simulink library "Simulation_lib"  (R2023b)
settings: Solver=VariableStepAuto  StartTime=0.0  StopTime=10.0  RelTol=1e-3
undefined symbols (not defined in the file): X, Y, Z
libraries: sm_lib x48, $bdroot x18, nesl_utility x16, fl_lib x15, ee_lib x3, simulink_extras x1
(part 3 of 3)

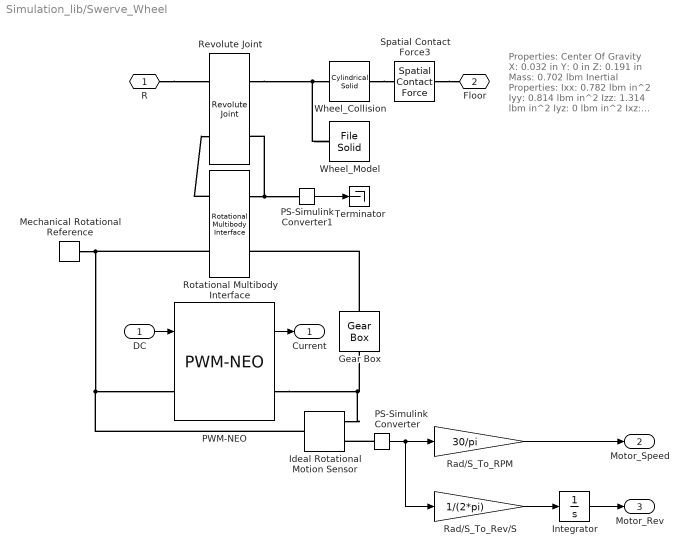
== system Simulation_lib/Swerve_Wheel ==
  note: Properties:
      | Center Of Gravity
      | X: 0.032 in
      | Y: 0 in
      | Z: 0.191 in
      | Mass: 0.702 lbm
      | Inertial Properties:
      | Ixx: 0.782 lbm in^2
      | Iyy: 0.814 lbm in^2
      | Izz: 1.314 lbm in^2
      | Iyz: 0 lbm in^2
      | Ixz: 0.004 lbm in^2
      | Ixy: 0 lbm in^2
      | Cut & Paste:
      | 0.702
      | [0.032 0 0.191]
      | [0.782 0.814 1.314]
      | [0 0.004 0]
  DC : Inport
  Gear Box : fl_lib/Mechanical/Mechanisms/Gear Box  ratio=8.14  t_in_specify=off  t_in_priority=None  t_in=0 N*m  t_in_nominal_specify=off  t_in_nominal_unit=N*m  t_in_nominal_value=1  t_out_specify=off  t_out_priority=None  t_out=0 N*m  t_out_nominal_specify=off  t_out_nominal_unit=N*m  t_out_nominal_value=1
  Ideal Rotational Motion Sensor : fl_lib/Mechanical/Mechanical Sensors/Ideal Rotational Motion Sensor  reference=foundation.enum.MeasurementReference.difference  acceleration_port=false  velocity_port=true  position_port=false  wrap_angle=false  offset=0 rad
      settings: InternalSimscapePortConfiguration="{\"Bottom\":[],\"Left\":[{\"id\":\"R\",\"label\":\"R\",\"type\":\"foundation.mechanical.rotational.rotational\"}],\"Right\":[{\"id\":\"C\",\"label\":\"C\",\"type\":\"foundation.mechanical.rotational.rotational\"},{\"id\":\"W\",\"label\":\"W\",\"type\":\"output\"}],\"Top\":[]}"
  Integrator : Integrator
  Mechanical Rotational Reference : fl_lib/Mechanical/Rotational Elements/Mechanical Rotational Reference
  PS-Simulink Converter : nesl_utility/PS-Simulink Converter  PhysicalDomain=network_engine_domain  SubClassName=ps_output  LeftPortType=input  RightPortType=output  PseudoPeriodic=off  Frequencies=[]  VectorFormat=inherit  Unit=inherit  AffineConversion=off
  PS-Simulink Converter1 : nesl_utility/PS-Simulink Converter  PhysicalDomain=network_engine_domain  SubClassName=ps_output  LeftPortType=input  RightPortType=output  PseudoPeriodic=off  Frequencies=[]  VectorFormat=inherit  Unit=inherit  AffineConversion=off
  PWM-NEO : $bdroot/PWM-NEO  SystemSampleTime=-1  VariantActivationTime=update diagram  AllowFlexibleInterface=on  Latency=0  AutoFrameSizeCalculation=off
  Rad/S_To_RPM : Gain  Gain=30/pi
  Rad/S_To_Rev/S : Gain  Gain=1/(2*pi)
  Revolute Joint : sm_lib/Joints/Revolute Joint  JointMode=Normal  SenseConstraintForce=off  SenseConstraintForceX=off  SenseConstraintForceY=off  SenseConstraintForceZ=off  SenseConstraintTorque=off  SenseConstraintTorqueX=off  SenseConstraintTorqueY=off  SenseConstraintTorqueZ=off  SenseTotalForce=off  SenseTotalForceX=off  SenseTotalForceY=off  SenseTotalForceZ=off  SenseTotalTorque=off  SenseTotalTorqueX=off  SenseTotalTorqueY=off  SenseTotalTorqueZ=off  CompositeWrenchDir=FollowerOnBase  CompositeWrenchFrame=BaseFrame  EquilibriumPosition=0  EquilibriumPositionUnits=deg  SpringStiffness=0  SpringStiffnessUnits=N*m/deg  DampingCoefficient=0  DampingCoefficientUnits=N*m/(deg/s)  TorqueActuationMode=InputTorque  MotionActuationMode=ComputedMotion  SensePosition=off  SenseVelocity=on  SenseAcceleration=off  SenseTorqueForce=off  SenseLowerLimitTorqueForce=off  SenseUpperLimitTorqueForce=off  LowerLimitSpecify=off  LowerLimitBound=-90  LowerLimitBoundUnits=deg  LowerLimitStiffness=1e4  LowerLimitStiffnessUnits=N*m/deg  LowerLimitDamping=10  LowerLimitDampingUnits=N*m/(deg/s)  LowerLimitTransitionRegionWidth=0.1  LowerLimitTransitionRegionWidthUnits=deg  UpperLimitSpecify=off  UpperLimitBound=90  UpperLimitBoundUnits=deg  UpperLimitStiffness=1e4  UpperLimitStiffnessUnits=N*m/deg  UpperLimitDamping=10  UpperLimitDampingUnits=N*m/(deg/s)  UpperLimitTransitionRegionWidth=0.1  UpperLimitTransitionRegionWidthUnits=deg  PositionTargetSpecify=off  PositionTargetPriority=High  PositionTargetValue=0  PositionTargetValueUnits=deg  VelocityTargetSpecify=off  VelocityTargetPriority=High  VelocityTargetValue=0  VelocityTargetValueUnits=deg/s
  Rotational Multibody Interface : fl_lib/Mechanical/Multibody Interfaces/Rotational Multibody Interface
  Spatial Contact Force3 : sm_lib/Forces and Torques/Spatial Contact Force  SenseContactBaseRotation=off  SenseContactBaseTranslation=off  CoefficientOfDynamicFriction=.45  CoefficientOfStaticFriction=.65  NormalDamping=1e3  NormalDampingUnits=N/(m/s)  SenseContactSignal=off  NormalStiffness=1e6  NormalStiffnessUnits=N/m  FrictionalCriticalVelocity=1e-3  FrictionalCriticalVelocityUnits=m/s  ZeroCrossDetectContactStartAndEnd=off  SenseContactFollowerRotation=off  SenseContactFollowerTranslation=off  FrictionType=SmoothStickSlip  SenseFrictionalForceMagnitude=off  SenseNormalForceMagnitude=off  NormalForceType=SmoothSpringDamper  SenseNormalVelocity=off  SensePenetrationDepth=off  SenseSeparationDistance=off  SenseTangentialVelocity=off  NormalTransitionRegionWidth=1e-4  NormalTransitionRegionWidthUnits=m
  Terminator : Terminator
  Wheel_Collision : sm_lib/Body Elements/Cylindrical Solid  GraphicAmbientColor=[0.15 0.15 0.15 1.0]  BasedOnType=Density  CenterOfMass=[0.032 0 0.191]  CenterOfMassUnits=in  GraphicDiffuseColor=[0.5 0.5 0.5]  CylinderLength=1.645  CylinderLengthUnits=in  CylinderRadius=2  CylinderRadiusUnits=in  Density=1000  DensityUnits=kg/m^3  DoExposeReferenceFrame=on  GraphicEmissiveColor=[0.0 0.0 0.0 1.0]  ExportEntireGeometry=on  SerializedFrames=<Frames/>  MarkerShape=Sphere  MarkerSize=10  GraphicType=None  InertiaType=Custom  Mass=0.702  MassUnits=lbm  MomentsOfInertia=[0.782 0.814 1.314]  MomentsOfInertiaUnits=lbm*in^2  GraphicOpacity=1.0  ProductsOfInertia=[0 0.004 0]  ProductsOfInertiaUnits=lbm*in^2  GraphicShininess=75  GraphicSpecularColor=[0.5 0.5 0.5 1.0]  GraphicVisPropType=SimpleVisualProperties
  Wheel_Model : sm_lib/Body Elements/File Solid  ExtGeomFileName=simulink\Reusable_Models\Simulation\Step_Models\wheel_Ass_mk4i.step  UnitType=FromFile  ExtGeomFileUnits=m  StepReaderType=HEX  ExportConvexHullGeometry=off  InertiaType=PointMass  Mass=0  MassUnits=lbm  CenterOfMass=[0.032 0 0.191]  CenterOfMassUnits=in  MomentsOfInertia=[0.782 0.814 1.314]  MomentsOfInertiaUnits=lbm*in^2  ProductsOfInertia=[0 0.004 0]  ProductsOfInertiaUnits=lbm*in^2  BasedOnType=DensityFromFile  Density=1000  DensityUnits=kg/m^3  DoExposeReferenceFrame=on  SerializedFrames=<Frames/>  GraphicType=FromGeometry  MarkerShape=Sphere  MarkerSize=10  GraphicVisPropType=SimpleVisualProperties  GraphicDiffuseColor=[0.4 0.4 1.0]  GraphicSpecularColor=[0.5 0.5 0.5 1.0]  GraphicAmbientColor=[0.15 0.15 0.15 1.0]  GraphicEmissiveColor=[0.0 0.0 0.0 1.0]  GraphicShininess=75  GraphicOpacity=1.0
  R : PMIOPort  Side=Left
  Floor : PMIOPort  Port=2  Side=Right
  Current : Outport
  Motor_Speed : Outport  Port=2
  Motor_Rev : Outport  Port=3  Unit=rev
  wires:
  PWM-NEO/1 -> Current/1
  DC/1 -> PWM-NEO/1
  PS-Simulink Converter/1 -> Rad/S_To_Rev/S/1, Rad/S_To_RPM/1
  Rad/S_To_RPM/1 -> Motor_Speed/1
  PS-Simulink Converter1/1 -> Terminator/1
  Rad/S_To_Rev/S/1 -> Integrator/1
  Integrator/1 -> Motor_Rev/1
  connections:
  Wheel_Model/RConn1 -- Wheel_Collision/RConn1 -- Revolute Joint/RConn1
  Wheel_Collision/LConn1 -- Spatial Contact Force3/LConn1
  Rotational Multibody Interface/LConn2 -- Mechanical Rotational Reference/LConn1 -- Ideal Rotational Motion Sensor/LConn1 -- PWM-NEO/LConn1
  Rotational Multibody Interface/RConn1 -- PS-Simulink Converter1/LConn1 -- Revolute Joint/RConn2
  PWM-NEO/RConn1 -- Ideal Rotational Motion Sensor/RConn1 -- Gear Box/LConn1
  Rotational Multibody Interface/LConn1 -- Revolute Joint/LConn2
  Gear Box/RConn1 -- Rotational Multibody Interface/RConn2
  R/RConn1 -- Revolute Joint/LConn1
  PS-Simulink Converter/LConn1 -- Ideal Rotational Motion Sensor/RConn2
  Spatial Contact Force3/RConn1 -- Floor/RConn1
